simulink model "model1"  (R2022a)
settings: Solver=VariableStepAuto  StartTime=0.0  StopTime=150  RelTol=1e-3
values from neighbouring files (symbols this model uses):
  A = [-9 1 ... (first row only)    [config.m]
  A_0g = [0          1 ... (first row only)    [config.m]
  A_m = [     0      1 ... (first row only)    [config.m]
  b = [3 ... (first row only)    [config.m]
  b_0g = [0 ... (first row only)    [config.m]
  C = [1 0]    [config.m]
  gamma = 0.5    [config.m]    (also in tasks.m = 1)
  K = H/M    [config.m]
settings Model: Creator=popov  LastModifiedBy=Vvlad
settings DebuggingCC: UnconnectedInputMsg=warning  UnconnectedOutputMsg=warning  UnconnectedLineMsg=warning
settings RTWCC: DLArmComputeVersion=19.05

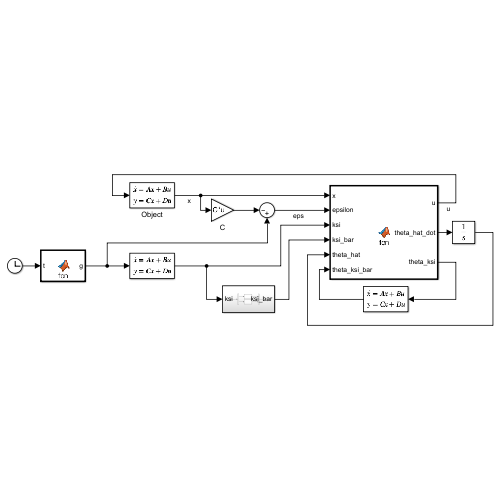
[thumbnail: Simulink's stored preview of the top-level diagram]
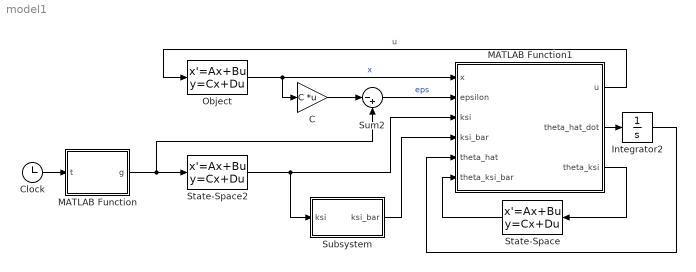
== system model1 ==
  C : Gain  Gain=C  Multiplication=Matrix(K*u)
  Clock : Clock
  Integrator2 : Integrator  InitialCondition=[0;0]
  MATLAB Function : MATLAB Function  TreatAsAtomicUnit=on
  MATLAB Function1 : MATLAB Function  TreatAsAtomicUnit=on
  Object : StateSpace  A=A  B=b  C=eye(2)  D=[0;0]  InitialCondition=0
  State-Space : StateSpace  A=A_m  B=b  C=C  D=0  InitialCondition=0
  State-Space2 : StateSpace  A=A_0g  B=b_0g  C=eye(2)  D=[0;0]  InitialCondition=0
  Subsystem : Subsystem
  Sum2 : Sum  Inputs=|-+
  wires:
  Clock/1 -> MATLAB Function/1(t)
  MATLAB Function/1(g) -> State-Space2/1, Sum2/2
  State-Space2/1 -> Subsystem/1(ksi), MATLAB Function1/3(ksi)
  MATLAB Function1/2(theta_hat_dot) -> Integrator2/1
  Integrator2/1 -> MATLAB Function1/5(theta_hat)
  MATLAB Function1/3(theta_ksi) -> State-Space/1
  State-Space/1 -> MATLAB Function1/6(theta_ksi_bar)
  Sum2/1 -> MATLAB Function1/2(epsilon)  "eps"
  Subsystem/1(ksi_bar) -> MATLAB Function1/4(ksi_bar)
  MATLAB Function1/1(u) -> Object/1  "u"
  Object/1 -> MATLAB Function1/1(x), C/1  "x"
  C/1 -> Sum2/1

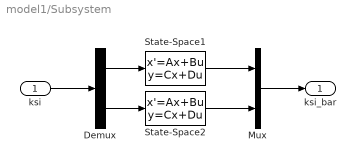
== system model1/Subsystem ==
  ksi : Inport
  Demux : Demux  Outputs=2
  Mux : Mux  Inputs=2
  State-Space1 : StateSpace  A=A_m  B=b  C=C  D=0  InitialCondition=0
  State-Space2 : StateSpace  A=A_m  B=b  C=C  D=0  InitialCondition=0
  ksi_bar : Outport
  wires:
  State-Space1/1 -> Mux/1
  Mux/1 -> ksi_bar/1
  Demux/2 -> State-Space2/1
  Demux/1 -> State-Space1/1
  State-Space2/1 -> Mux/2
  ksi/1 -> Demux/1

== matlab function model1/MATLAB Function1 ==
  data: x input; epsilon input; u output; ksi input; ksi_bar input; theta_hat input; theta_hat_dot output; K parameter; theta_ksi output; theta_ksi_bar input; gamma parameter
function [u,theta_hat_dot, theta_ksi] = fcn(x, epsilon, ksi, ksi_bar, theta_hat, K, theta_ksi_bar, gamma)

theta_ksi = theta_hat'*ksi;
epsilon_hat = epsilon - theta_hat'*ksi_bar + theta_ksi_bar;
theta_hat_dot = gamma*ksi_bar*epsilon_hat;
u = -K*x + theta_hat'*ksi;

== matlab function model1/MATLAB Function ==
  data: t input; g output
function g = fcn(t)

g = 6*cos(3*t+3);
